simulink model "Simulacion"  (Simulink 10.1)
settings: Solver=ode45  StartTime=0.0  StopTime=1000  RelTol=1e-3  EnableMultiTasking=on
settings Model: Creator=Helbert  LastModifiedBy=leidy
settings DataIOCC: LimitDataPoints=on  SignalLoggingSaveFormat=ModelDataLogs
settings OptimizationCC: InitFltsAndDblsToZero=on
settings DebuggingCC: SaveWithParameterizedLinksMsg=none  SignalResolutionControl=TryResolveAllWithWarning  SolverPrmCheckMsg=warning  MultiTaskDSMMsg=warning  MultiTaskCondExecSysMsg=none
settings GRTTargetCC: TargetFcnLib=ansi_tfl_tmw.mat

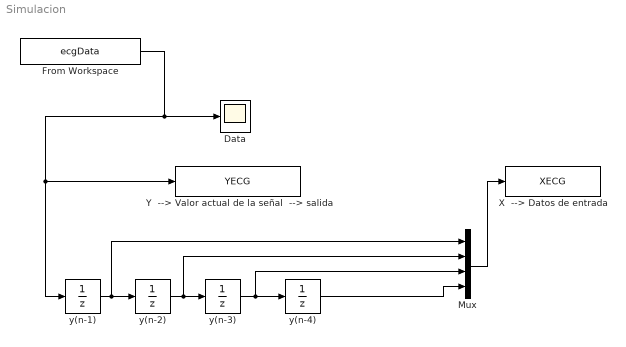
== system Simulacion ==
  Data : Scope
  From Workspace : FromWorkspace  VariableName=ecgData  SampleTime=1  ZeroCross=off
  Mux : Mux
  X  --> Datos de entrada : ToWorkspace  VariableName=XECG  SampleTime=1
  Y  --> Valor actual de la señal  --> salida : ToWorkspace  VariableName=YECG  SampleTime=1
  y(n-1) : UnitDelay  HasFrameUpgradeWarning=on
  y(n-2) : UnitDelay  HasFrameUpgradeWarning=on
  y(n-3) : UnitDelay  HasFrameUpgradeWarning=on
  y(n-4) : UnitDelay  HasFrameUpgradeWarning=on
  wires:
  From Workspace/1 -> y(n-1)/1, Y  --> Valor actual de la señal  --> salida/1, Data/1
  y(n-1)/1 -> y(n-2)/1, Mux/1
  y(n-2)/1 -> y(n-3)/1, Mux/2
  Mux/1 -> X  --> Datos de entrada/1
  y(n-3)/1 -> y(n-4)/1, Mux/3
  y(n-4)/1 -> Mux/4
